simulink model "MOD_5_Counter"  (R2020b)
settings: Solver=VariableStepAuto  StartTime=0.0  StopTime=10.0  RelTol=1e-3
settings Model: Creator=Shree  LastModifiedBy=Shree

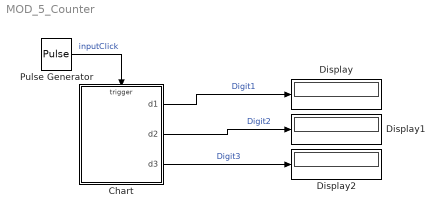
== system MOD_5_Counter ==
  Chart : Stateflow chart  TreatAsAtomicUnit=on
  Display : Display
  Display1 : Display
  Display2 : Display
  Pulse Generator : DiscretePulseGenerator  PulseType=Time based  Period=0.1  PulseWidth=0.5
  wires:
  Chart/2(d2) -> Display1/1  "Digit2"
  Chart/3(d3) -> Display2/1  "Digit3"
  Chart/1(d1) -> Display/1  "Digit1"
  Pulse Generator/1 -> Chart/Trigger  "inputClick"

== stateflow chart MOD_5_Counter/Chart ==
  settings: executeAtInitialization=1
  state A
    state Digit1 [parallel]
      settings: executionOrder=1
      state one
        en: d1 = 1;
      state two
        en: d1 = 2;
      state zero
        en: d1 = 0;
      state three
        en: d1 = 3;
      state four
        en: d1 = 4;
      A.Digit1.one -> A.Digit1.two : inputClick
      A.Digit1.zero -> A.Digit1.one : inputClick
      A.Digit1.two -> A.Digit1.three : inputClick
      (default) -> A.Digit1.zero
      A.Digit1.four -> A.Digit1.zero : inputClick /{inc2;}
      A.Digit1.three -> A.Digit1.four : inputClick
    state Digit2 [parallel]
      settings: executionOrder=2
      state one
        en: d2 = 1;
      state two
        en: d2 = 2;
      state zero
        en: d2 = 0;
      state three
        en: d2 = 3;
      state four
        en: d2 = 4;
      A.Digit2.one -> A.Digit2.two : inc2
      A.Digit2.zero -> A.Digit2.one : inc2
      A.Digit2.two -> A.Digit2.three : inc2
      (default) -> A.Digit2.zero
      A.Digit2.four -> A.Digit2.zero : inc2/{inc3;}
      A.Digit2.three -> A.Digit2.four : inc2
    state Digit3 [parallel]
      settings: executionOrder=3
      state one
        en: d3 = 1;
      state two
        en: d3 = 2;
      state zero
        en: d3 = 0;
      state three
        en: d3 = 3;
      state four
        en: d3 = 4;
      A.Digit3.one -> A.Digit3.two : inc3
      A.Digit3.zero -> A.Digit3.one : inc3
      A.Digit3.two -> A.Digit3.three : inc3
      (default) -> A.Digit3.zero
      A.Digit3.four -> A.Digit3.zero : inc3
      A.Digit3.three -> A.Digit3.four : inc3
  (default) -> A
  data: d1 output; d2 output; d3 output
  events: inputClick input RISING_EDGE_EVENT; inc2 local FUNCTION_CALL_EVENT; inc3 local FUNCTION_CALL_EVENT
